simulink model "stb_disc"  (Simulink 5.0)
settings: Solver=ode45  StartTime=t_init  StopTime=t_final  RelTol=1e-3
values from neighbouring files (symbols this model uses):
  A = axes('FontSize',fs)    [axesprop.m]    (also in seshft.m = [A zeros(Arows,Bcols-Acols)])
  B = -B    [left_prm.m]    (also in myc2d.m = num(first_nz:length(num)); seshft.m = [B zeros(Brows,Acols-Bcols)])
  C = [eye(Fbcols) zeros(Fbcols,Scols-Fbcols)]    [left_prm.m]    (also in seshft.m = [A)
undefined symbols (not defined in the file or in its folder): D, gamma, N_var, Rc, Sc, st, Tc, Ts, zk
libraries: simulink x2
settings Model: Creator=kannan  LastModifiedBy=kannan  ExtModeAutoUpdateStatusClock=off

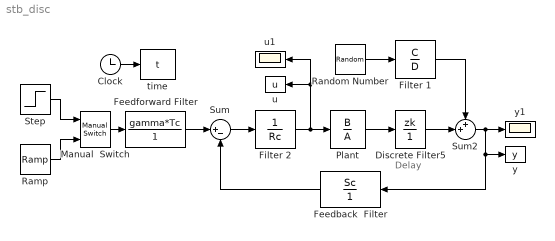
== system stb_disc ==
  note: Delay
  " Filter 2" : DiscreteFilter  Numerator=1  Denominator=Rc  SampleTime=Ts
  Clock : Clock
      settings: Decimation=10
  Discrete Filter5 : DiscreteFilter  Numerator=zk  Denominator=1  SampleTime=Ts
  Feedback  Filter : DiscreteFilter  Orientation=left  Numerator=Sc  Denominator=1  SampleTime=Ts
  Feedforward Filter : DiscreteFilter  Numerator=gamma*Tc  Denominator=1  SampleTime=Ts
  Filter 1 : DiscreteFilter  Numerator=C  Denominator=D  SampleTime=Ts
  Manual  Switch : simulink/Signal Routing/Manual Switch  sw=0  action=0
  Plant : DiscreteFilter  Numerator=B  Denominator=A  SampleTime=Ts
  Ramp : simulink/Sources/Ramp  slope=1  start=t_init  X0=0
  Random Number : RandomNumber  Variance=N_var  SampleTime=Ts
  Step : Step  Time=0  After=st  SampleTime=Ts
  Sum : Sum  Inputs=|+-  SaturateOnIntegerOverflow=on
  Sum2 : Sum  Inputs=++|  SaturateOnIntegerOverflow=on
  time : ToWorkspace  VariableName=t  SampleTime=Ts  SaveFormat=Array
  u : ToWorkspace  VariableName=u  SampleTime=Ts  SaveFormat=Array
  u1 : Scope
      settings: YMin=0  YMax=1.4
  y : ToWorkspace  VariableName=y  SampleTime=Ts  SaveFormat=Array
  y1 : Scope
      settings: YMin=0  YMax=1.2
  wires:
  Feedforward Filter/1 -> Sum/1
  Feedback  Filter/1 -> Sum/2
  Clock/1 -> time/1
  Plant/1 -> Discrete Filter5/1
  Discrete Filter5/1 -> Sum2/2
  Filter 1/1 -> Sum2/1
  Random Number/1 -> Filter 1/1
  Sum2/1 -> y1/1, Feedback  Filter/1, y/1
  Sum/1 -> " Filter 2"/1
  " Filter 2"/1 -> Plant/1, u1/1, u/1
  Manual  Switch/1 -> Feedforward Filter/1
  Step/1 -> Manual  Switch/1
  Ramp/1 -> Manual  Switch/2
